simulink model "wmr"  (R2021b)
settings: Solver=VariableStepAuto  StartTime=0.0  StopTime=10.0  RelTol=1e-3
settings Model: Creator=xuans  LastModifiedBy=xuans

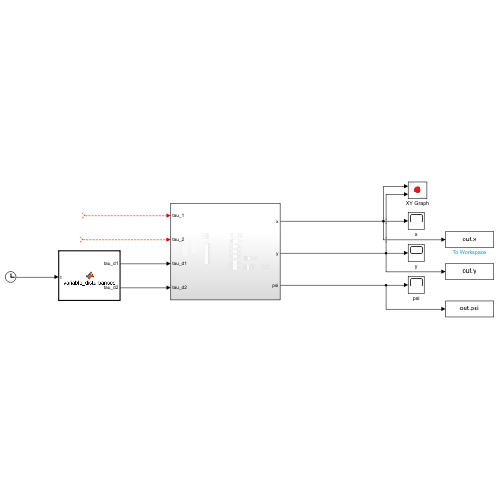
[thumbnail: Simulink's stored preview of the top-level diagram]
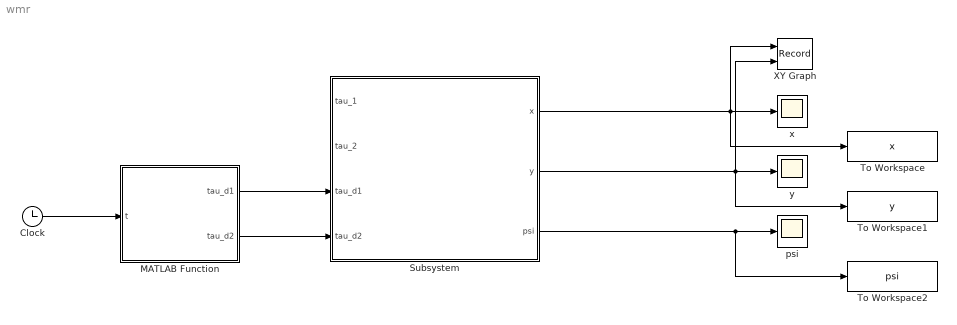
== system wmr ==
  Clock : Clock
  MATLAB Function : MATLAB Function  TreatAsAtomicUnit=on
  Subsystem : Subsystem
  To Workspace : ToWorkspace  VariableName=x  SaveFormat=Timeseries  SampleTime=-1
  To Workspace1 : ToWorkspace  VariableName=y  SaveFormat=Timeseries  SampleTime=-1
  To Workspace2 : ToWorkspace  VariableName=psi  SaveFormat=Timeseries  SampleTime=-1
  XY Graph : Record  FileSettingsInternal="{\"entries\":[{\"content\":{\"excelSettings\":{\"content\":{},\"type\":\"Streamout.ExcelSettings\"}},\"type\":\"Streamout.FileSettingStorage\",\"uuid\":\"08cd0689-42de-4b4e-938f-1b053c6d5192\"}],\"packageUris\":[\"http://schema.mathworks.com/mf0/streamout_blocks/R2020a\"],\"version\":\"1.0\"}"  Layout=[1 1]  SignalsInternal="{\"entries\":[{\"content\":{\"signals\":[{\"content\":{\"blockPath\":[\"wmr/XY Graph\"],\"channel\":[],\"dimensions\":[1],\"domain\":\"wmr/XY Graph\",\"lineColor\":\"#a2142f\",\"plots\":[1],\"port\":1,\"sid\":[],\"signalID\":17,\"signalName\":\"XY Graph:1\"},\"type\":\"RecordBlkView.Signal\",\"uuid\":\"5ff1d324-96d5-491c-9e9f-f8ab79186796\"},{\"content\":{\"blockPath\":[\"wmr/XY Graph\"],\"channel\":[],\"dimensions\":[1],\"domain\":\"wmr/XY Graph\",\"lineColor\":\"#139fff\",\"plots\":[1],\"port\":2,\"sid\":[],\"signalID\":20,\"signalName\":\"XY Graph:2\"},\"type\":\"RecordBlkView.Signal\",\"uuid\":\"905abbf6-86fa-4ecf-b766-ba2f6adc6666\"}]},\"type\":\"RecordBlkView.InputSignals\",\"uuid\":\"b5fdf117-84ec-41c8-9457-9b3fa2f8500d\"}],\"packageUris\":[\"http://schema.mathworks.com/mf0/streamout_blocks/R2020a\"],\"version\":\"1.0\"}"  VisualizationBindings="{\"xyplotplugin\":{\"info\":[{\"series\":[{\"bindingParametersList\":[{\"parameter\":\"X-Axis\",\"signalID\":17,\"signalName\":\"XY Graph:1\"},{\"parameter\":\"Y-Axis\",\"signalID\":20,\"signalName\":\"XY Graph:2\"}],\"seriesID\":49855}],\"subplotID\":1}]}}"  CompatibilityTag=XY
  psi : Scope
  x : Scope
  y : Scope
  wires:
  Clock/1 -> MATLAB Function/1(t)
  MATLAB Function/1(tau_d1) -> Subsystem/3(tau_d1)
  MATLAB Function/2(tau_d2) -> Subsystem/4(tau_d2)
  Subsystem/1(x) -> x/1, To Workspace/1, XY Graph/1
  Subsystem/2(y) -> To Workspace1/1, XY Graph/2, y/1
  Subsystem/3(psi) -> To Workspace2/1, psi/1
  ? -> Subsystem/1(tau_1)
  ? -> Subsystem/2(tau_2)

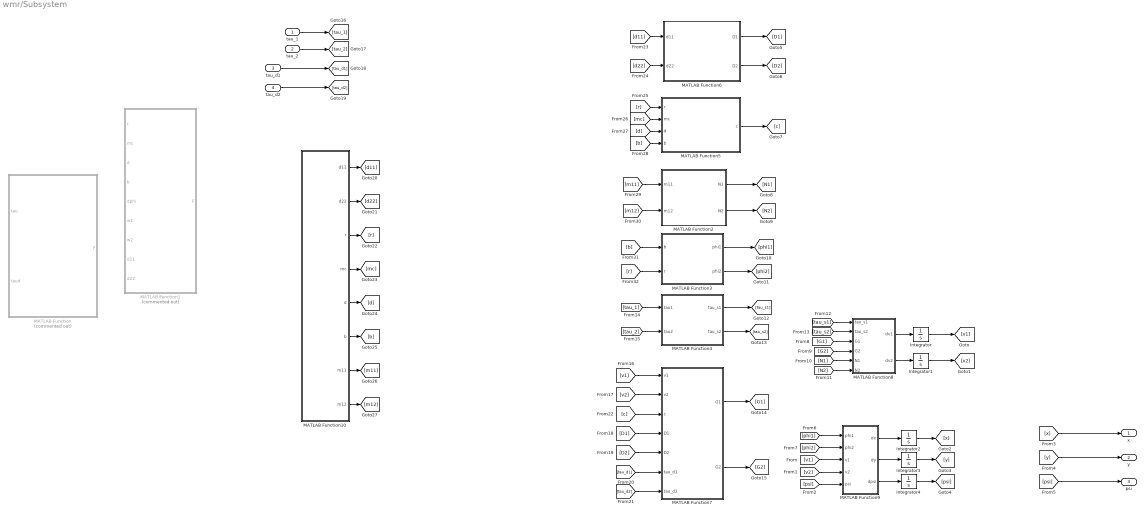
== system wmr/Subsystem ==
  tau_1 : Inport
  tau_2 : Inport  Port=2
  tau_d1 : Inport  Port=3
  tau_d2 : Inport  Port=4
  Integrator{,1..4} (5 alike) : Integrator
  MATLAB Function : MATLAB Function  Commented=on  TreatAsAtomicUnit=on
  MATLAB Function1 : MATLAB Function  Commented=on  TreatAsAtomicUnit=on
  MATLAB Function10 : MATLAB Function  TreatAsAtomicUnit=on
  MATLAB Function2 : MATLAB Function  TreatAsAtomicUnit=on
  MATLAB Function3 : MATLAB Function  TreatAsAtomicUnit=on
  MATLAB Function4 : MATLAB Function  TreatAsAtomicUnit=on
  MATLAB Function5 : MATLAB Function  TreatAsAtomicUnit=on
  MATLAB Function6 : MATLAB Function  TreatAsAtomicUnit=on
  MATLAB Function7 : MATLAB Function  TreatAsAtomicUnit=on
  MATLAB Function8 : MATLAB Function  TreatAsAtomicUnit=on
  MATLAB Function9 : MATLAB Function  TreatAsAtomicUnit=on
  x : Outport
  y : Outport  Port=2
  psi : Outport  Port=3
  wires:
  [x] -> x/1
  tau_1/1 -> [tau_1]
  MATLAB Function8/1(dv1) -> Integrator/1
  MATLAB Function8/2(dv2) -> Integrator1/1
  Integrator/1 -> [v1]
  Integrator1/1 -> [v2]
  [v2] -> MATLAB Function9/4(v2)
  [v1] -> MATLAB Function9/3(v1)
  MATLAB Function9/3(dpsi) -> Integrator4/1
  MATLAB Function9/2(dy) -> Integrator3/1
  MATLAB Function9/1(dx) -> Integrator2/1
  Integrator2/1 -> [x]
  Integrator3/1 -> [y]
  Integrator4/1 -> [psi]
  [psi] -> MATLAB Function9/5(psi)
  [y] -> y/1
  [psi] -> psi/1
  MATLAB Function6/1(D1) -> [D1]
  MATLAB Function6/2(D2) -> [D2]
  MATLAB Function5/1(c) -> [c]
  MATLAB Function2/1(N1) -> [N1]
  MATLAB Function2/2(N2) -> [N2]
  MATLAB Function3/1(phi1) -> [phi1]
  MATLAB Function3/2(phi2) -> [phi2]
  MATLAB Function4/1(tau_s1) -> [tau_s1]
  MATLAB Function4/2(tau_s2) -> [tau_s2]
  MATLAB Function7/1(G1) -> [G1]
  MATLAB Function7/2(G2) -> [G2]
  [phi2] -> MATLAB Function9/2(phi2)
  [phi1] -> MATLAB Function9/1(phi1)
  [G1] -> MATLAB Function8/3(G1)
  [G2] -> MATLAB Function8/4(G2)
  [N1] -> MATLAB Function8/5(N1)
  [N2] -> MATLAB Function8/6(N2)
  [tau_s1] -> MATLAB Function8/1(tau_s1)
  [tau_s2] -> MATLAB Function8/2(tau_s2)
  tau_2/1 -> [tau_2]
  [tau_1] -> MATLAB Function4/1(tau1)
  [tau_2] -> MATLAB Function4/2(tau2)
  [v1] -> MATLAB Function7/1(v1)
  [v2] -> MATLAB Function7/2(v2)
  [D1] -> MATLAB Function7/4(D1)
  [D2] -> MATLAB Function7/5(D2)
  tau_d2/1 -> [tau_d2]
  tau_d1/1 -> [tau_d1]
  [tau_d1] -> MATLAB Function7/6(tau_d1)
  [tau_d2] -> MATLAB Function7/7(tau_d2)
  [c] -> MATLAB Function7/3(c)
  MATLAB Function10/1(d11) -> [d11]
  MATLAB Function10/2(d22) -> [d22]
  MATLAB Function10/3(r) -> [r]
  MATLAB Function10/4(mc) -> [mc]
  MATLAB Function10/5(d) -> [d]
  MATLAB Function10/6(b) -> [b]
  MATLAB Function10/7(m11) -> [m11]
  MATLAB Function10/8(m12) -> [m12]
  [d11] -> MATLAB Function6/1(d11)
  [d22] -> MATLAB Function6/2(d22)
  [r] -> MATLAB Function5/1(r)
  [mc] -> MATLAB Function5/2(mc)
  [d] -> MATLAB Function5/3(d)
  [b] -> MATLAB Function5/4(b)
  [m11] -> MATLAB Function2/1(m11)
  [m12] -> MATLAB Function2/2(m12)
  [b] -> MATLAB Function3/1(b)
  [r] -> MATLAB Function3/2(r)

== matlab function wmr/Subsystem/MATLAB Function9 ==
  data: phi1 input; dx output; phi2 input; v1 input; v2 input; psi input; dy output; dpsi output
function [dx,dy,dpsi] = fcn(phi1,phi2,v1,v2,psi)

dx=phi1*v1*cos(psi);
dy=phi1*v1*sin(psi);
dpsi=phi2*v2;

== matlab function wmr/Subsystem/MATLAB Function10 ==
  data: d11 output; d22 output; r output; mc output; d output; b output; m11 output; m12 output
function [d11,d22, r, mc, d, b, m11, m12] = constant

d11=10;
d22=10;
r=0.15;
b=0.75;
d=0.3;
mc=30;
%tau_M=50;  %maximum of control torques
mw=1;
Ic=15.625;
Iw=0.005;
Im=mw*(r^2)+2*(Ic/r);  % 没找到。。scispace说的
I0=mc*d^2+2*mw*b^2+Ic+2*Im;
m11=((r^2)/(4*b^2))*((mc+2*mw)*(b^2)+I0)+Iw;
m12=((r^2)/(4*b^2))*((mc+2*mw)*(b^2)-I0);

== matlab function wmr/MATLAB Function ==
  data: t input; tau_d1 output; tau_d2 output
function [tau_d1,tau_d2] = variable_disturbances(t)

y = u;

== matlab function wmr/Subsystem/MATLAB Function1 ==
  data: r input; F output; mc input; d input; b input; dphi input; w1 input; w2 input; d11 input; d22 input
function F = Fq(r,mc,d,b,dphi,w1,w2,d11,d22)



F1=-(r^2*mc*d)/2b))*dphi*w2-d11*w1;
F2=(r^2*mc*d)/2b))*dphi*w1-d22*w2;


F=[F1,F2]';

== matlab function wmr/Subsystem/MATLAB Function ==
  data: tau input; y output; taud input
function y = fcn(tau,taud)



F1=-((r^2*mc*d)/2b)*dphi*w2-d11*w1;
F2=((r^2*mc*d)/2b)*dphi*w1-d22*w2;


y = u;

== matlab function wmr/Subsystem/MATLAB Function2 ==
  data: m11 input; N1 output; m12 input; N2 output
function [N1,N2] = constant_N(m11,m12)

N1=2*(m11+m12);
N2=2*(m11-m12);

== matlab function wmr/Subsystem/MATLAB Function3 ==
  data: b input; phi1 output; r input; phi2 output
function [phi1,phi2] = constant_phi(b,r)

phi1=r;
phi2=r/b;

== matlab function wmr/Subsystem/MATLAB Function4 ==
  data: tau1 input; tau_s1 output; tau2 input; tau_s2 output
function [tau_s1,tau_s2] = variable_tau_s(tau1,tau2)
tau_s1=tau1+tau2;
tau_s2=tau1-tau2;

== matlab function wmr/Subsystem/MATLAB Function5 ==
  data: r input; c output; mc input; d input; b input
function c = constant_c(r,mc,d,b)

c=((r^3)*mc*d)/(2*b^2);

== matlab function wmr/Subsystem/MATLAB Function6 ==
  data: d11 input; D1 output; d22 input; D2 output
function [D1,D2] = constant_damping_terms(d11,d22)

D1=d11+d22;
D2=d11-d22;

== matlab function wmr/Subsystem/MATLAB Function7 ==
  data: G1 output; v1 input; v2 input; c input; D1 input; D2 input; tau_d1 input; tau_d2 input; G2 output
function [G1,G2] = variable_G(v1,v2,c,D1,D2,tau_d1,tau_d2)

G1=-c*v2^2-D1*v1-D2*v2+tau_d1+tau_d2;
G2=c*v1*v2-D2*v1-D1*v2+tau_d1-tau_d2;

== matlab function wmr/Subsystem/MATLAB Function8 ==
  data: tau_s1 input; dv1 output; tau_s2 input; G1 input; G2 input; dv2 output; N1 input; N2 input
function [dv1,dv2]  = fuc_v(tau_s1,tau_s2,G1,G2,N1,N2)
dv1=(tau_s1+G1)/N1;
dv2=(tau_s2+G2)/N2;
